simulink model "Model3"  (R2022b)
settings: Solver=VariableStepAuto  StartTime=0.0  StopTime=60  RelTol=1e-3
values from neighbouring files (symbols this model uses):
  K_A = 0.2    [script2.m]
  K_B = 2.2    [script2.m]
libraries: cstblocks x2
settings Model: Creator=Sahil Gaurkar  LastModifiedBy=Sahil Gaurkar

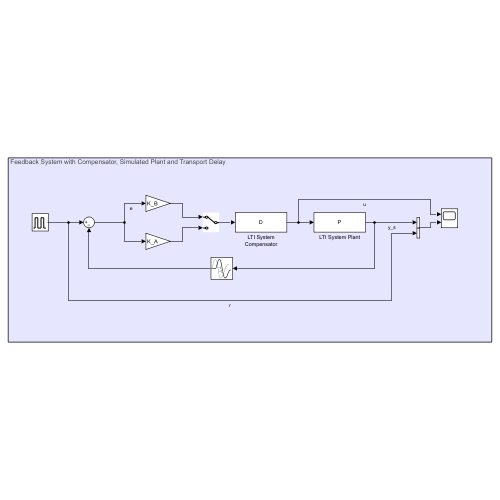
[thumbnail: Simulink's stored preview of the top-level diagram]
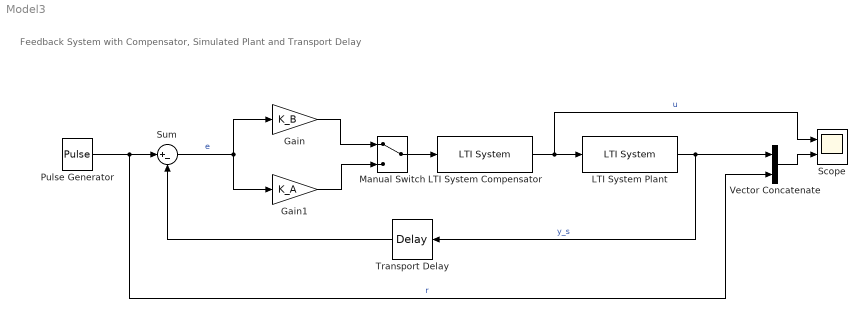
== system Model3 ==
  note: Feedback System with Compensator, Simulated Plant and Transport Delay
  Gain : Gain  Gain=K_B
  Gain1 : Gain  Gain=K_A
  LTI System Compensator : cstblocks/LTI System  sys=D  IC=[]
  LTI System Plant : cstblocks/LTI System  sys=P  IC=[]
  Manual Switch : ManualSwitch
  Pulse Generator : DiscretePulseGenerator  PulseType=Time based  Period=10  PulseWidth=50
  Scope : Scope  NumInputPorts=2
  Sum : Sum  Inputs=|+-
  Transport Delay : TransportDelay  DelayTime=0.025
  Vector Concatenate : Concatenate
  wires:
  Sum/1 -> Gain1/1, Gain/1  "e"
  Vector Concatenate/1 -> Scope/2
  LTI System Compensator/1 -> Scope/1, LTI System Plant/1  "u"
  Gain1/1 -> Manual Switch/2
  Manual Switch/1 -> LTI System Compensator/1
  LTI System Plant/1 -> Vector Concatenate/1, Transport Delay/1  "y_s"
  Gain/1 -> Manual Switch/1
  Pulse Generator/1 -> Vector Concatenate/2, Sum/1  "r"
  Transport Delay/1 -> Sum/2
